simulink model "Enacba_zasuka_volana"  (R2020b)
settings: Solver=VariableStepAuto  StartTime=0.0  StopTime=1  RelTol=1e-3
libraries: simulink_extras x3, vehdynlibsteering x2
settings Model: Creator=lugh8  LastModifiedBy=lugh8

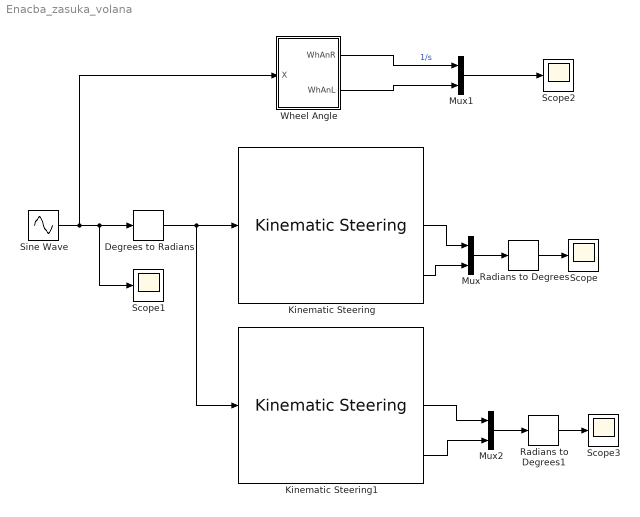
== system Enacba_zasuka_volana ==
  Degrees to Radians : simulink_extras/Transformations/Degrees to Radians
  Kinematic Steering : vehdynlibsteering/Kinematic Steering  StrgType=Rack and pinion  StrgRatioType=Constant  Loc=Front  NrmlFctr=0.01  TrckWdth=1.098  WhlBase=1.524  Db=0  StrgRng=3.66  StrgAngBpts="[-6.2832   -5.0265   -3.7699   -2.5133   -1.2566         0    1.2566    2.5133    3.7699    5.0265    6.2832]"  StrgRatioTbl=|  StrgRatio=100  StrgArmLngth=0.08088  RckCsLngth=0.29  TieRodLngth=0.458282  D=0.03  PnnRadius=0.019  PnnRadiusTbl="[0.0055    0.0055    0.0056    0.0057    0.0058    0.0057    0.0057    0.0057    0.0056    0.0055    0.0055]"  RodLngth=0.1  ParaArmLngth=0.9  aMode=2
      | [13.5000   13.3750   13.2500   13.1250   13.0000   13.0000   13.0000   13.1250   13.2500   13.3750   13.5000
      | ]
  Kinematic Steering1 : vehdynlibsteering/Kinematic Steering  StrgType=Ackerman  StrgRatioType=Constant  Loc=Front  NrmlFctr=0.01  TrckWdth=1.098  WhlBase=1.524  Db=0  StrgRng=3.66  StrgAngBpts="[-6.2832   -5.0265   -3.7699   -2.5133   -1.2566         0    1.2566    2.5133    3.7699    5.0265    6.2832]"  StrgRatioTbl=|  StrgRatio=4  StrgArmLngth=0.08088  RckCsLngth=0.29  TieRodLngth=0.458282  D=0.03  PnnRadius=0.019  PnnRadiusTbl="[0.0055    0.0055    0.0056    0.0057    0.0058    0.0057    0.0057    0.0057    0.0056    0.0055    0.0055]"  RodLngth=0.1  ParaArmLngth=0.9  aMode=2
      | [13.5000   13.3750   13.2500   13.1250   13.0000   13.0000   13.0000   13.1250   13.2500   13.3750   13.5000
      | ]
  Mux : Mux  Inputs=2
  Mux1 : Mux  Inputs=2
  Mux2 : Mux  Inputs=2
  Radians to Degrees : simulink_extras/Transformations/Radians to Degrees
  Radians to Degrees1 : simulink_extras/Transformations/Radians to Degrees
  Scope{,1..3} (4 alike) : Scope
  Sine Wave : Sin  Amplitude=105  Frequency=10  SampleTime=0
  Wheel Angle : MATLAB Function  TreatAsAtomicUnit=on
  wires:
  Kinematic Steering/2 -> Mux/1
  Kinematic Steering/3 -> Mux/2
  Mux/1 -> Radians to Degrees/1
  Sine Wave/1 -> Wheel Angle/1(X), Scope1/1, Degrees to Radians/1
  Degrees to Radians/1 -> Kinematic Steering1/1, Kinematic Steering/1
  Radians to Degrees/1 -> Scope/1
  Wheel Angle/2(WhAnL) -> Mux1/2
  Wheel Angle/1(WhAnR) -> Mux1/1  "1/s"
  Mux1/1 -> Scope2/1
  Radians to Degrees1/1 -> Scope3/1
  Mux2/1 -> Radians to Degrees1/1
  Kinematic Steering1/3 -> Mux2/2
  Kinematic Steering1/2 -> Mux2/1

== matlab function Enacba_zasuka_volana/Wheel Angle ==
  data: X input; WhAnR output; WhAnL output
function [WhAnR,WhAnL] = fcn(X)
%#codegen

if X >= 0
    WhAnL = -4E-11*X^6 + 8E-9*X^5 - 6E-7*X^4 + 3E-5*X^3 - 4E-4*X^2 + 0.2045*X + 0.0034;
    WhAnR = -1E-10*X^6 + 3E-8*X^5 - 3E-6*X^4 + 1E-4*X^3 - 0.0015*X^2 + 0.2149*X - 0.0102;
else
    WhAnR = -4E-11*X^6 + 8E-9*X^5 - 6E-7*X^4 + 3E-5*X^3 - 4E-4*X^2 + 0.2045*X + 0.0034;
    WhAnL = -1E-10*X^6 + 3E-8*X^5 - 3E-6*X^4 + 1E-4*X^3 - 0.0015*X^2 + 0.2149*X - 0.0102;
end
